simulink model "controller_simulation"  (R2024a)
settings: Solver=ode45  StartTime=0.0  StopTime=35  FixedStep=0.01  MaxStep=0.01  RelTol=1e-3
values from neighbouring files (symbols this model uses):
  Kd = diag([40,  40,  40,  40])    [initialize.m]
  Kp = diag([500, 500, 500, 500])    [initialize.m]
  q_init = traj.Vitridat(2:5, 1)    [initialize.m]
settings Model: Creator=hason  LastModifiedBy=hason
settings DataIOCC: OutputOption=SpecifiedOutputTimes  OutputTimes=[0:0.01:35]

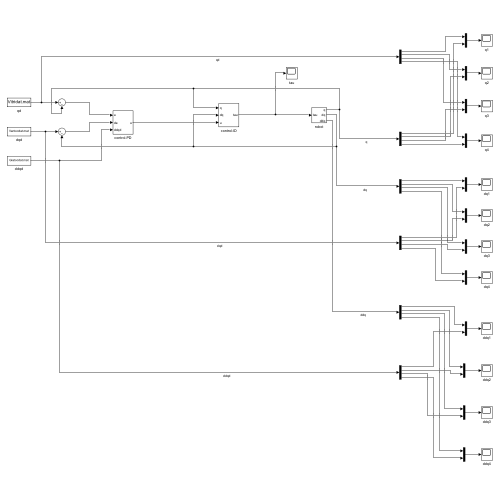
[thumbnail: Simulink's stored preview of the top-level diagram]
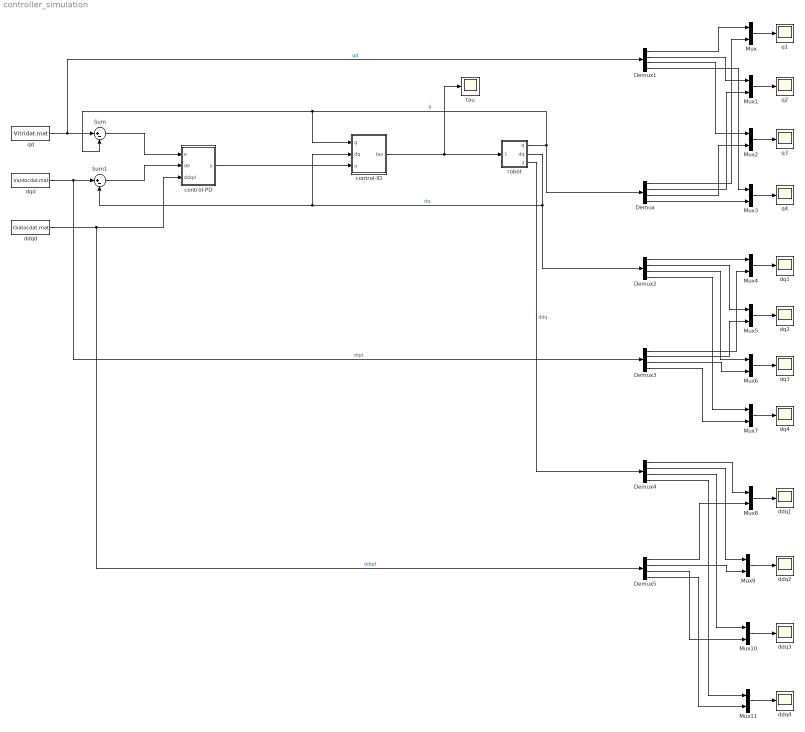
== system controller_simulation ==
  Demux{,1..5} (6 alike) : Demux
  Mux{,1..11} (12 alike) : Mux  Inputs=2
  Sum : Sum  Inputs=|+-
  Sum1 : Sum  Inputs=|+-
  control-ID : Subsystem
  control-PD : Subsystem
  ddq{1..4} (4 alike) : Scope
  ddqd : FromFile  FileName=Giatocdat.mat  SampleTime=0.01  ExtrapolationBeforeFirstDataPoint=Hold first value  InterpolationWithinTimeRange=Zero order hold  ExtrapolationAfterLastDataPoint=Ground value
  dq{1..4} (4 alike) : Scope
  dqd : FromFile  FileName=Vantocdat.mat  SampleTime=0.01  ExtrapolationBeforeFirstDataPoint=Hold first value  ExtrapolationAfterLastDataPoint=Ground value
  q{1..4} (4 alike) : Scope
  qd : FromFile  FileName=Vitridat.mat  SampleTime=0.01  ExtrapolationBeforeFirstDataPoint=Hold first value  ExtrapolationAfterLastDataPoint=Hold last value
  robot : Subsystem
  tau : Scope
  wires:
  qd/1 -> Sum/1, Demux1/1  "qd"
  dqd/1 -> Demux3/1, Sum1/1  "dqd"
  Sum/1 -> control-PD/1(e)
  Sum1/1 -> control-PD/2(de)
  ddqd/1 -> Demux5/1, control-PD/3(ddqd)  "ddqd"
  robot/1(q) -> Demux/1, control-ID/1(q), Sum/2  "q"
  control-PD/1(u) -> control-ID/3(u)
  control-ID/1(tau) -> tau/1, robot/1(tau)
  Demux1/1 -> Mux/1
  Mux/1 -> q1/1
  Mux3/1 -> q4/1
  Mux2/1 -> q3/1
  Mux1/1 -> q2/1
  Demux/1 -> Mux/2
  Demux1/2 -> Mux1/1
  Demux/2 -> Mux1/2
  Demux1/3 -> Mux2/1
  Demux/3 -> Mux2/2
  Demux1/4 -> Mux3/1
  Demux/4 -> Mux3/2
  robot/2(dq) -> Demux2/1, control-ID/2(dq), Sum1/2  "dq"
  Mux4/1 -> dq1/1
  Demux2/1 -> Mux4/1
  Demux3/1 -> Mux4/2
  Mux5/1 -> dq2/1
  Mux6/1 -> dq3/1
  Mux7/1 -> dq4/1
  Demux2/2 -> Mux5/1
  Demux3/2 -> Mux5/2
  Demux2/3 -> Mux6/1
  Demux3/3 -> Mux6/2
  Demux2/4 -> Mux7/1
  Demux3/4 -> Mux7/2
  robot/3(ddq) -> Demux4/1  "ddq"
  Mux8/1 -> ddq1/1
  Mux9/1 -> ddq2/1
  Mux10/1 -> ddq3/1
  Mux11/1 -> ddq4/1
  Demux4/1 -> Mux8/1
  Demux4/2 -> Mux9/1
  Demux4/3 -> Mux10/1
  Demux4/4 -> Mux11/1
  Demux5/1 -> Mux8/2
  Demux5/2 -> Mux9/2
  Demux5/3 -> Mux10/2
  Demux5/4 -> Mux11/2

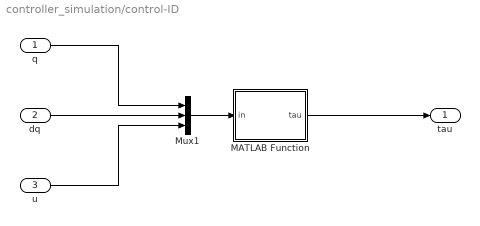
== system controller_simulation/control-ID ==
  q : Inport
  dq : Inport  Port=2
  u : Inport  Port=3
  MATLAB Function : MATLAB Function  TreatAsAtomicUnit=on
  Mux1 : Mux  Inputs=3
  tau : Outport
  wires:
  Mux1/1 -> MATLAB Function/1(in)
  q/1 -> Mux1/1
  MATLAB Function/1(tau) -> tau/1
  u/1 -> Mux1/3
  dq/1 -> Mux1/2

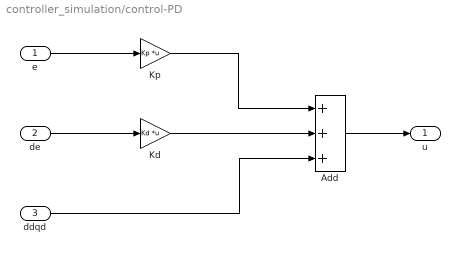
== system controller_simulation/control-PD ==
  e : Inport
  de : Inport  Port=2
  ddqd : Inport  Port=3
  Add : Sum  Inputs=+++
  Kd : Gain  Gain=Kd  Multiplication=Matrix(K*u)
  Kp : Gain  Gain=Kp  Multiplication=Matrix(K*u)
  u : Outport
  wires:
  Add/1 -> u/1
  Kp/1 -> Add/1
  ddqd/1 -> Add/3
  Kd/1 -> Add/2
  de/1 -> Kd/1
  e/1 -> Kp/1

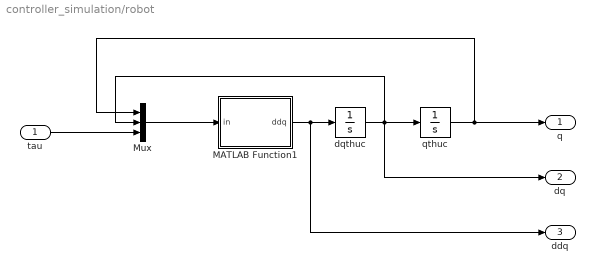
== system controller_simulation/robot ==
  tau : Inport
  MATLAB Function1 : MATLAB Function  TreatAsAtomicUnit=on
  Mux : Mux  Inputs=3
  dqthuc : Integrator  InitialCondition=[0; 0; 0; 0]
  qthuc : Integrator  InitialCondition=q_init
  q : Outport
  dq : Outport  Port=2
  ddq : Outport  Port=3
  wires:
  qthuc/1 -> q/1, Mux/1
  tau/1 -> Mux/3
  dqthuc/1 -> dq/1, qthuc/1, Mux/2
  Mux/1 -> MATLAB Function1/1(in)
  MATLAB Function1/1(ddq) -> ddq/1, dqthuc/1

== matlab function controller_simulation/control-ID/MATLAB Function ==
  data: in input; tau output; p parameter
function tau = ID_controller(in, p)
    % Input: in = [q1; q2; q3; q4; dq1; dq2; dq3; dq4; u1; u2; u3; u4]
    % Output: tau = [tau1; tau2; tau3; tau4]

    % --- 0. Khởi tạo kích thước đầu ra (Bắt buộc để cổng ra hiện số 4) ---
    tau = zeros(4,1);
    
    % --- 1. Tách biến từ input Simulink (Đổi sang dq để tránh trùng tên) ---
    q1  = in(1);  q2  = in(2);  q3  = in(3);  q4  = in(4);
    dq1 = in(5);  dq2 = in(6);  dq3 = in(7);  dq4 = in(8);
    u   = in(9:12); % u là tín hiệu gia tốc lệnh (Size 4x1)
    
    % --- 2. Khai báo biến global ---
    g = p.g; a2 = p.a2; d3 = p.d3; d4 = p.d4;
    m1 = p.m1; m2 = p.m2; m3 = p.m3; m4 = p.m4;
    xc1 = p.xc1; xc2 = p.xc2; xc3 = p.xc3; xc4 = p.xc4; % THÊM p.xc1 vào đây
    yc1 = p.yc1; yc3 = p.yc3; yc4 = p.yc4;              % Đã có p.yc1
    zc2 = p.zc2; zc3 = p.zc3; zc4 = p.zc4;
    Ixx3 = p.Ixx3; Ixx4 = p.Ixx4; Iyy2 = p.Iyy2; Iyy3 = p.Iyy3; Iyy4 = p.Iyy4; 
    Izz1 = p.Izz1; Izz3 = p.Izz3; Izz4 = p.Izz4;
    Ixy3 = p.Ixy3; Ixy4 = p.Ixy4; Ixz3 = p.Ixz3; Ixz4 = p.Ixz4; Iyz3 = p.Iyz3; Iyz4 = p.Iyz4;
    
    % --- 3. Tính toán Ma trận M, C, G (Copy từ robot_model) ---
    Cq1 = cos(q1); Sq1 = sin(q1);
    Cq3 = cos(q3); Sq3 = sin(q3);
    Cq4 = cos(q4); Sq4 = sin(q4);
    
    M = zeros(4,4);
    
    M(1,1) = (((-xc4^2+yc4^2)*m4+Ixx4)*Cq4^2+2*Sq4*(m4*xc4*yc4-Ixy4)*Cq4+Iyy4*Sq4^2+(d4+zc4)^2*m4+m3*zc3^2+Ixx3)*Cq3^2+2*(((-xc4*(d4+zc4)*m4+Ixz4)*Cq4+(yc4*(d4+zc4)*m4-Iyz4)*Sq4-m3*xc3*zc3+Ixz3)*Sq3+((d4+zc4)*m4+m3*zc3)*a2)*Cq3+(m3*xc3^2+m4*yc4^2+Izz3+Izz4)*Sq3^2-2*a2*(xc4*m4*Cq4-yc4*Sq4*m4+xc3*m3)*Sq3+2*d3*m4*yc4*Cq4+2*d3*m4*xc4*Sq4+(a2^2+d3^2+xc4^2)*m4+(m2+m3)*a2^2+2*a2*m2*xc2+(d3+yc3)^2*m3+(xc2^2+zc2^2)*m2+(xc1^2+yc1^2)*m1+Iyy2+Izz1;
    M(1,2) = 0;
    M(1,3) = (2*(-m4*xc4*yc4+Ixy4)*Cq4^2+(((-xc4^2+yc4^2)*m4+Ixx4-Iyy4)*Sq4-d3*m4*xc4)*Cq4+d3*yc4*Sq4*m4-d3*m3*xc3+m4*xc4*yc4-m3*xc3*yc3+Ixy3-Ixy4)*Cq3-((yc4*(d4+zc4)*m4-Iyz4)*Cq4+(xc4*(d4+zc4)*m4-Ixz4)*Sq4+d3*(d4+zc4)*m4+d3*m3*zc3+m3*yc3*zc3-Iyz3)*Sq3;
    M(1,4) = ((-xc4*(d4+zc4)*m4+Ixz4)*Cq4-(-yc4*(d4+zc4)*m4+Iyz4)*Sq4)*Cq3-m4*(-d3*yc4*Sq3+a2*xc4)*Cq4+(d3*m4*xc4*Sq4+(xc4^2+yc4^2)*m4+Izz4)*Sq3+a2*m4*yc4*Sq4;
    M(2,1) = 0; M(2,2) = m2+m3+m4;
    M(2,3) = ((d4+zc4)*m4+m3*zc3)*Cq3-Sq3*(xc4*m4*Cq4-yc4*Sq4*m4+xc3*m3);
    M(2,4) = -(Sq4*xc4+Cq4*yc4)*Cq3*m4;
    M(3,1) = M(1,3); M(3,2) = M(2,3);
    M(3,3) = (m4*xc4^2+Iyy4)*Cq4^2+2*Sq4*(-m4*xc4*yc4+Ixy4)*Cq4+(m4*yc4^2+Ixx4)*Sq4^2+(d4+zc4)^2*m4+m3*xc3^2+m3*zc3^2+Iyy3;
    M(3,4) = (-yc4*(d4+zc4)*m4+Iyz4)*Cq4-(xc4*(d4+zc4)*m4-Ixz4)*Sq4;
    M(4,1) = M(1,4); M(4,2) = M(2,4); M(4,3) = M(3,4);
    M(4,4) = Izz4+(xc4^2+yc4^2)*m4;
    
    C = zeros(4,4);
    
    C(1,1) = (dq4*(m4*xc4*yc4-Ixy4)*Cq4^2+(((xc4^2-yc4^2)*m4-Ixx4+Iyy4)*dq4*Sq4-dq3*(xc4*(d4+zc4)*m4-Ixz4))*Cq4-dq4*(m4*xc4*yc4-Ixy4)*Sq4^2+dq3*(yc4*(d4+zc4)*m4-Iyz4)*Sq4-dq3*(m3*xc3*zc3-Ixz3))*Cq3^2+((dq3*((xc4^2-yc4^2)*m4-Ixx4)*Cq4^2+(-2*dq3*(m4*xc4*yc4-Ixy4)*Sq4+(yc4*(d4+zc4)*m4-Iyz4)*dq4)*Cq4-Iyy4*Sq4^2*dq3+(xc4*(d4+zc4)*m4-Ixz4)*dq4*Sq4+((yc4+zc4+d4)*(yc4-zc4-d4)*m4+(xc3^2-zc3^2)*m3-Ixx3+Izz3+Izz4)*dq3)*Sq3-a2*dq3*(xc4*m4*Cq4-yc4*Sq4*m4+xc3*m3))*Cq3+((xc4*(d4+zc4)*m4-Ixz4)*Cq4+(-yc4*(d4+zc4)*m4+Iyz4)*Sq4+m3*xc3*zc3-Ixz3)*dq3*Sq3^2+a2*(yc4*m4*dq4*Cq4+xc4*Sq4*m4*dq4-dq3*((d4+zc4)*m4+m3*zc3))*Sq3+d3*m4*dq4*(Cq4*xc4-Sq4*yc4);
    C(1,3) = -((xc4*(d4+zc4)*m4-Ixz4)*Cq4+(-yc4*(d4+zc4)*m4+Iyz4)*Sq4+m3*xc3*zc3-Ixz3)*dq1*Cq3^2+1/2*(2*(((xc4^2-yc4^2)*m4-Ixx4)*Cq4^2-2*Sq4*(m4*xc4*yc4-Ixy4)*Cq4-Iyy4*Sq4^2+(yc4+zc4+d4)*(yc4-zc4-d4)*m4+(xc3^2-zc3^2)*m3-Ixx3+Izz3+Izz4)*dq1*Sq3-((xc4^2-yc4^2)*m4-Ixx4+Iyy4)*dq4*Cq4^2+2*(2*dq4*(m4*xc4*yc4-Ixy4)*Sq4+(-a2*xc4*dq1+(-(d4+zc4)*dq3+dq4*d3)*yc4)*m4+Iyz4*dq3)*Cq4+((xc4^2-yc4^2)*m4-Ixx4+Iyy4)*dq4*Sq4^2+2*((a2*yc4*dq1+(-(d4+zc4)*dq3+dq4*d3)*xc4)*m4+Ixz4*dq3)*Sq4+(-2*d3*(d4+zc4)*dq3+dq4*(xc4^2+yc4^2))*m4-2*a2*m3*dq1*xc3+2*(-zc3*(d3+yc3)*m3+Iyz3)*dq3+Izz4*dq4)*Cq3-Sq3*(-((xc4*(d4+zc4)*m4-Ixz4)*Cq4+(-yc4*(d4+zc4)*m4+Iyz4)*Sq4+m3*xc3*zc3-Ixz3)*dq1*Sq3-2*dq3*(m4*xc4*yc4-Ixy4)*Cq4^2-dq3*(((xc4^2-yc4^2)*m4-Ixx4+Iyy4)*Sq4+d3*m4*xc4)*Cq4+Sq4*d3*m4*dq3*yc4+(a2*(d4+zc4)*dq1+xc4*yc4*dq3)*m4+a2*m3*dq1*zc3-(xc3*(d3+yc3)*m3-Ixy3+Ixy4)*dq3);
    C(1,4) = (Cq4^2*(m4*xc4*yc4-Ixy4)+((xc4^2-yc4^2)*m4-Ixx4+Iyy4)*Sq4*Cq4-Sq4^2*(m4*xc4*yc4-Ixy4))*dq1*Cq3^2+1/2*(-((xc4^2-yc4^2)*m4-Ixx4+Iyy4)*dq3*Cq4^2+2*(2*dq3*(m4*xc4*yc4-Ixy4)*Sq4+(yc4*(d4+zc4)*m4-Iyz4)*dq1*Sq3+yc4*(d3*dq3+dq4*(d4+zc4))*m4-Iyz4*dq4)*Cq4+((xc4^2-yc4^2)*m4-Ixx4+Iyy4)*dq3*Sq4^2+2*((xc4*(d4+zc4)*m4-Ixz4)*dq1*Sq3+xc4*(d3*dq3+dq4*(d4+zc4))*m4-Ixz4*dq4)*Sq4+dq3*(Izz4+(xc4^2+yc4^2)*m4))*Cq3+m4*(((a2*dq1*yc4+d3*dq4*xc4)*Sq3+a2*yc4*dq4+xc4*d3*dq1)*Cq4+((a2*dq1*xc4-d3*dq4*yc4)*Sq3+a2*xc4*dq4-yc4*d3*dq1)*Sq4);
    C(2,3) = (yc4*m4*dq4*Cq4+xc4*Sq4*m4*dq4-dq3*((d4+zc4)*m4+m3*zc3))*Sq3+Cq3*dq3*(-xc4*m4*Cq4+yc4*Sq4*m4-xc3*m3);
    C(2,4) = m4*(dq4*(-Cq4*xc4+Sq4*yc4)*Cq3+dq3*(Sq4*xc4+Cq4*yc4)*Sq3);
    C(3,1) = ((xc4*(d4+zc4)*m4-Ixz4)*Cq4+(-yc4*(d4+zc4)*m4+Iyz4)*Sq4+m3*xc3*zc3-Ixz3)*dq1*Cq3^2+1/2*(-2*(((xc4^2-yc4^2)*m4-Ixx4)*Cq4^2-2*Sq4*(m4*xc4*yc4-Ixy4)*Cq4-Iyy4*Sq4^2+(yc4+zc4+d4)*(yc4-zc4-d4)*m4+(xc3^2-zc3^2)*m3-Ixx3+Izz3+Izz4)*dq1*Sq3-((xc4^2-yc4^2)*m4-Ixx4+Iyy4)*dq4*Cq4^2+2*(2*dq4*(m4*xc4*yc4-Ixy4)*Sq4+a2*m4*dq1*xc4)*Cq4+((xc4^2-yc4^2)*m4-Ixx4+Iyy4)*dq4*Sq4^2-2*Sq4*a2*m4*dq1*yc4+2*a2*m3*dq1*xc3-(Izz4+(xc4^2+yc4^2)*m4)*dq4)*Cq3+(-((xc4*(d4+zc4)*m4-Ixz4)*Cq4+(-yc4*(d4+zc4)*m4+Iyz4)*Sq4+m3*xc3*zc3-Ixz3)*dq1*Sq3-(xc4*(d4+zc4)*m4-Ixz4)*dq4*Cq4+(yc4*(d4+zc4)*m4-Iyz4)*dq4*Sq4+dq1*a2*((d4+zc4)*m4+m3*zc3))*Sq3;
    C(3,3) = -1/2*(((xc4^2-yc4^2)*m4-Ixx4+Iyy4)*sin(2*q4)+2*cos(2*q4)*(m4*xc4*yc4-Ixy4))*dq4;
    C(3,4) = (dq1*(-m4*xc4^2+Ixx4-Iyy4)*Cq3+2*dq3*(-m4*xc4*yc4+Ixy4))*Cq4^2+((-2*dq1*(-m4*xc4*yc4+Ixy4)*Cq3+dq3*((-xc4^2+yc4^2)*m4+Ixx4-Iyy4))*Sq4-(dq4+Sq3*dq1)*(xc4*(d4+zc4)*m4-Ixz4))*Cq4-Cq3*Sq4^2*m4*dq1*yc4^2+(yc4*(d4+zc4)*m4-Iyz4)*(dq4+Sq3*dq1)*Sq4-1/2*dq1*(Ixx4-Iyy4+Izz4)*Cq3-dq3*(-m4*xc4*yc4+Ixy4);
    C(4,1) = ((-m4*xc4*yc4+Ixy4)*Cq4^2+((-xc4^2+yc4^2)*m4+Ixx4-Iyy4)*Sq4*Cq4+Sq4^2*(m4*xc4*yc4-Ixy4))*dq1*Cq3^2+1/2*(-((-xc4^2+yc4^2)*m4+Ixx4-Iyy4)*dq3*Cq4^2+2*(-2*dq3*(m4*xc4*yc4-Ixy4)*Sq4-(yc4*(d4+zc4)*m4-Iyz4)*dq1*Sq3)*Cq4+((-xc4^2+yc4^2)*m4+Ixx4-Iyy4)*dq3*Sq4^2-2*(xc4*(d4+zc4)*m4-Ixz4)*Sq3*dq1*Sq4+dq3*(Izz4+(xc4^2+yc4^2)*m4))*Cq3+(((xc4*(d4+zc4)*dq3-a2*yc4*dq1)*m4-Ixz4*dq3)*Sq3-d3*m4*dq1*xc4)*Cq4-Sq4*(((yc4*(d4+zc4)*dq3+a2*xc4*dq1)*m4-Iyz4*dq3)*Sq3-d3*m4*dq1*yc4);
    C(4,3) = (-dq1*(-m4*xc4^2+Ixx4-Iyy4)*Cq3-2*dq3*(-m4*xc4*yc4+Ixy4))*Cq4^2+((2*dq1*(-m4*xc4*yc4+Ixy4)*Cq3-dq3*((-xc4^2+yc4^2)*m4+Ixx4-Iyy4))*Sq4+(xc4*(d4+zc4)*m4-Ixz4)*dq1*Sq3)*Cq4+Cq3*Sq4^2*m4*dq1*yc4^2-dq1*(yc4*(d4+zc4)*m4-Iyz4)*Sq3*Sq4+1/2*dq1*(Ixx4-Iyy4+Izz4)*Cq3+dq3*(-m4*xc4*yc4+Ixy4);
    
    G = zeros(4,1);
    G(2,1) = g*(m2+m3+m4);
    G(3,1) = g*(((d4+zc4)*m4+m3*zc3)*Cq3-Sq3*(xc4*m4*Cq4-yc4*Sq4*m4+xc3*m3));
    G(4,1) = -m4*(Sq4*xc4+Cq4*yc4)*Cq3*g;
    
    % --- 4. Luật điều khiển IDPD (Computed Torque) ---
    dq_vector = [dq1; dq2; dq3; dq4]; % Vector cột 4x1
    
    % Phép toán: (4x4)*(4x1) + (4x4)*(4x1) + (4x1) = (4x1)
    tau = M * u + C * dq_vector + G;
end

== matlab function controller_simulation/robot/MATLAB Function1 ==
  data: in input; ddq output; p parameter
function ddq = fcn(in, p)
    % Input: in = [q1, q2, q3, q4, dq1, dq2, dq3, dq4, tau1, tau2, tau3, tau4]
    
    % --- 0. Khởi tạo kích thước đầu ra (Bắt buộc để cổng ra hiện số 4) ---
    ddq = zeros(4,1);
    
    % --- 1. Tách tín hiệu (Đổi sang dq để tránh trùng tên biến) ---
    q = in(1:4); 
    dq_vec = in(5:8); % Vector vận tốc khớp thực tế (4x1)
    tau = in(9:12);   % Vector mô-men xoắn từ bộ điều khiển đưa vào (4x1)
    
    q1=q(1);   q2=q(2);   q3=q(3);   q4=q(4);
    dq1=dq_vec(1); dq2=dq_vec(2); dq3=dq_vec(3); dq4=dq_vec(4);
    
    % --- 2. Khai báo biến toàn cục ---
    g = p.g; a2 = p.a2; d3 = p.d3; d4 = p.d4;
    m1 = p.m1; m2 = p.m2; m3 = p.m3; m4 = p.m4;
    xc1 = p.xc1; xc2 = p.xc2; xc3 = p.xc3; xc4 = p.xc4; % THÊM p.xc1 vào đây
    yc1 = p.yc1; yc3 = p.yc3; yc4 = p.yc4;              % Đã có p.yc1
    zc2 = p.zc2; zc3 = p.zc3; zc4 = p.zc4;
    Ixx3 = p.Ixx3; Ixx4 = p.Ixx4; Iyy2 = p.Iyy2; Iyy3 = p.Iyy3; Iyy4 = p.Iyy4; 
    Izz1 = p.Izz1; Izz3 = p.Izz3; Izz4 = p.Izz4;
    Ixy3 = p.Ixy3; Ixy4 = p.Ixy4; Ixz3 = p.Ixz3; Ixz4 = p.Ixz4; Iyz3 = p.Iyz3; Iyz4 = p.Iyz4;
    
    % --- 3. Tính toán Ma trận M, C, G ---
    Cq1 = cos(q1); Sq1 = sin(q1); Cq3 = cos(q3); Sq3 = sin(q3); Cq4 = cos(q4); Sq4 = sin(q4);
    
    % ---- Ma tran khoi luong M(q) ----
    M = zeros(4,4);
    M(1,1) = (((-xc4^2+yc4^2)*m4+Ixx4)*Cq4^2+2*Sq4*(m4*xc4*yc4-Ixy4)*Cq4+Iyy4*Sq4^2+(d4+zc4)^2*m4+m3*zc3^2+Ixx3)*Cq3^2+2*(((-xc4*(d4+zc4)*m4+Ixz4)*Cq4+(yc4*(d4+zc4)*m4-Iyz4)*Sq4-m3*xc3*zc3+Ixz3)*Sq3+((d4+zc4)*m4+m3*zc3)*a2)*Cq3+(m3*xc3^2+m4*yc4^2+Izz3+Izz4)*Sq3^2-2*a2*(xc4*m4*Cq4-yc4*Sq4*m4+xc3*m3)*Sq3+2*d3*m4*yc4*Cq4+2*d3*m4*xc4*Sq4+(a2^2+d3^2+xc4^2)*m4+(m2+m3)*a2^2+2*a2*m2*xc2+(d3+yc3)^2*m3+(xc2^2+zc2^2)*m2+(xc1^2+yc1^2)*m1+Iyy2+Izz1;
    M(1,2) = 0;
    M(1,3) = (2*(-m4*xc4*yc4+Ixy4)*Cq4^2+(((-xc4^2+yc4^2)*m4+Ixx4-Iyy4)*Sq4-d3*m4*xc4)*Cq4+d3*yc4*Sq4*m4-d3*m3*xc3+m4*xc4*yc4-m3*xc3*yc3+Ixy3-Ixy4)*Cq3-((yc4*(d4+zc4)*m4-Iyz4)*Cq4+(xc4*(d4+zc4)*m4-Ixz4)*Sq4+d3*(d4+zc4)*m4+d3*m3*zc3+m3*yc3*zc3-Iyz3)*Sq3;
    M(1,4) = ((-xc4*(d4+zc4)*m4+Ixz4)*Cq4-(-yc4*(d4+zc4)*m4+Iyz4)*Sq4)*Cq3-m4*(-d3*yc4*Sq3+a2*xc4)*Cq4+(d3*m4*xc4*Sq4+(xc4^2+yc4^2)*m4+Izz4)*Sq3+a2*m4*yc4*Sq4;
    M(2,1) = 0;
    M(2,2) = m2+m3+m4;
    M(2,3) = ((d4+zc4)*m4+m3*zc3)*Cq3-Sq3*(xc4*m4*Cq4-yc4*Sq4*m4+xc3*m3);
    M(2,4) = -(Sq4*xc4+Cq4*yc4)*Cq3*m4;
    M(3,1) = M(1,3);
    M(3,2) = M(2,3);
    M(3,3) = (m4*xc4^2+Iyy4)*Cq4^2+2*Sq4*(-m4*xc4*yc4+Ixy4)*Cq4+(m4*yc4^2+Ixx4)*Sq4^2+(d4+zc4)^2*m4+m3*xc3^2+m3*zc3^2+Iyy3;
    M(3,4) = (-yc4*(d4+zc4)*m4+Iyz4)*Cq4-(xc4*(d4+zc4)*m4-Ixz4)*Sq4;
    M(4,1) = M(1,4);
    M(4,2) = M(2,4);
    M(4,3) = M(3,4);
    M(4,4) = Izz4+(xc4^2+yc4^2)*m4;
    
    % ---- Ma tran Coriolis C(q,dq) ----
    C = zeros(4,4);
    C(1,1) = (dq4*(m4*xc4*yc4-Ixy4)*Cq4^2+(((xc4^2-yc4^2)*m4-Ixx4+Iyy4)*dq4*Sq4-dq3*(xc4*(d4+zc4)*m4-Ixz4))*Cq4-dq4*(m4*xc4*yc4-Ixy4)*Sq4^2+dq3*(yc4*(d4+zc4)*m4-Iyz4)*Sq4-dq3*(m3*xc3*zc3-Ixz3))*Cq3^2+((dq3*((xc4^2-yc4^2)*m4-Ixx4)*Cq4^2+(-2*dq3*(m4*xc4*yc4-Ixy4)*Sq4+(yc4*(d4+zc4)*m4-Iyz4)*dq4)*Cq4-Iyy4*Sq4^2*dq3+(xc4*(d4+zc4)*m4-Ixz4)*dq4*Sq4+((yc4+zc4+d4)*(yc4-zc4-d4)*m4+(xc3^2-zc3^2)*m3-Ixx3+Izz3+Izz4)*dq3)*Sq3-a2*dq3*(xc4*m4*Cq4-yc4*Sq4*m4+xc3*m3))*Cq3+((xc4*(d4+zc4)*m4-Ixz4)*Cq4+(-yc4*(d4+zc4)*m4+Iyz4)*Sq4+m3*xc3*zc3-Ixz3)*dq3*Sq3^2+a2*(yc4*m4*dq4*Cq4+xc4*Sq4*m4*dq4-dq3*((d4+zc4)*m4+m3*zc3))*Sq3+d3*m4*dq4*(Cq4*xc4-Sq4*yc4);
    C(1,2) = 0;
    C(1,3) = -((xc4*(d4+zc4)*m4-Ixz4)*Cq4+(-yc4*(d4+zc4)*m4+Iyz4)*Sq4+m3*xc3*zc3-Ixz3)*dq1*Cq3^2+1/2*(2*(((xc4^2-yc4^2)*m4-Ixx4)*Cq4^2-2*Sq4*(m4*xc4*yc4-Ixy4)*Cq4-Iyy4*Sq4^2+(yc4+zc4+d4)*(yc4-zc4-d4)*m4+(xc3^2-zc3^2)*m3-Ixx3+Izz3+Izz4)*dq1*Sq3-((xc4^2-yc4^2)*m4-Ixx4+Iyy4)*dq4*Cq4^2+2*(2*dq4*(m4*xc4*yc4-Ixy4)*Sq4+(-a2*xc4*dq1+(-(d4+zc4)*dq3+dq4*d3)*yc4)*m4+Iyz4*dq3)*Cq4+((xc4^2-yc4^2)*m4-Ixx4+Iyy4)*dq4*Sq4^2+2*((a2*yc4*dq1+(-(d4+zc4)*dq3+dq4*d3)*xc4)*m4+Ixz4*dq3)*Sq4+(-2*d3*(d4+zc4)*dq3+dq4*(xc4^2+yc4^2))*m4-2*a2*m3*dq1*xc3+2*(-zc3*(d3+yc3)*m3+Iyz3)*dq3+Izz4*dq4)*Cq3-Sq3*(-((xc4*(d4+zc4)*m4-Ixz4)*Cq4+(-yc4*(d4+zc4)*m4+Iyz4)*Sq4+m3*xc3*zc3-Ixz3)*dq1*Sq3-2*dq3*(m4*xc4*yc4-Ixy4)*Cq4^2-dq3*(((xc4^2-yc4^2)*m4-Ixx4+Iyy4)*Sq4+d3*m4*xc4)*Cq4+Sq4*d3*m4*dq3*yc4+(a2*(d4+zc4)*dq1+xc4*yc4*dq3)*m4+a2*m3*dq1*zc3-(xc3*(d3+yc3)*m3-Ixy3+Ixy4)*dq3);
    C(1,4) = (Cq4^2*(m4*xc4*yc4-Ixy4)+((xc4^2-yc4^2)*m4-Ixx4+Iyy4)*Sq4*Cq4-Sq4^2*(m4*xc4*yc4-Ixy4))*dq1*Cq3^2+1/2*(-((xc4^2-yc4^2)*m4-Ixx4+Iyy4)*dq3*Cq4^2+2*(2*dq3*(m4*xc4*yc4-Ixy4)*Sq4+(yc4*(d4+zc4)*m4-Iyz4)*dq1*Sq3+yc4*(d3*dq3+dq4*(d4+zc4))*m4-Iyz4*dq4)*Cq4+((xc4^2-yc4^2)*m4-Ixx4+Iyy4)*dq3*Sq4^2+2*((xc4*(d4+zc4)*m4-Ixz4)*dq1*Sq3+xc4*(d3*dq3+dq4*(d4+zc4))*m4-Ixz4*dq4)*Sq4+dq3*(Izz4+(xc4^2+yc4^2)*m4))*Cq3+m4*(((a2*dq1*yc4+d3*dq4*xc4)*Sq3+a2*yc4*dq4+xc4*d3*dq1)*Cq4+((a2*dq1*xc4-d3*dq4*yc4)*Sq3+a2*xc4*dq4-yc4*d3*dq1)*Sq4);
    C(2,1) = 0;
    C(2,2) = 0;
    C(2,3) = (yc4*m4*dq4*Cq4+xc4*Sq4*m4*dq4-dq3*((d4+zc4)*m4+m3*zc3))*Sq3+Cq3*dq3*(-xc4*m4*Cq4+yc4*Sq4*m4-xc3*m3);
    C(2,4) = m4*(dq4*(-Cq4*xc4+Sq4*yc4)*Cq3+dq3*(Sq4*xc4+Cq4*yc4)*Sq3);
    C(3,1) = ((xc4*(d4+zc4)*m4-Ixz4)*Cq4+(-yc4*(d4+zc4)*m4+Iyz4)*Sq4+m3*xc3*zc3-Ixz3)*dq1*Cq3^2+1/2*(-2*(((xc4^2-yc4^2)*m4-Ixx4)*Cq4^2-2*Sq4*(m4*xc4*yc4-Ixy4)*Cq4-Iyy4*Sq4^2+(yc4+zc4+d4)*(yc4-zc4-d4)*m4+(xc3^2-zc3^2)*m3-Ixx3+Izz3+Izz4)*dq1*Sq3-((xc4^2-yc4^2)*m4-Ixx4+Iyy4)*dq4*Cq4^2+2*(2*dq4*(m4*xc4*yc4-Ixy4)*Sq4+a2*m4*dq1*xc4)*Cq4+((xc4^2-yc4^2)*m4-Ixx4+Iyy4)*dq4*Sq4^2-2*Sq4*a2*m4*dq1*yc4+2*a2*m3*dq1*xc3-(Izz4+(xc4^2+yc4^2)*m4)*dq4)*Cq3+(-((xc4*(d4+zc4)*m4-Ixz4)*Cq4+(-yc4*(d4+zc4)*m4+Iyz4)*Sq4+m3*xc3*zc3-Ixz3)*dq1*Sq3-(xc4*(d4+zc4)*m4-Ixz4)*dq4*Cq4+(yc4*(d4+zc4)*m4-Iyz4)*dq4*Sq4+dq1*a2*((d4+zc4)*m4+m3*zc3))*Sq3;
    C(3,2) = 0;
    C(3,3) = -1/2*(((xc4^2-yc4^2)*m4-Ixx4+Iyy4)*sin(2*q4)+2*cos(2*q4)*(m4*xc4*yc4-Ixy4))*dq4;
    C(3,4) = (dq1*(-m4*xc4^2+Ixx4-Iyy4)*Cq3+2*dq3*(-m4*xc4*yc4+Ixy4))*Cq4^2+((-2*dq1*(-m4*xc4*yc4+Ixy4)*Cq3+dq3*((-xc4^2+yc4^2)*m4+Ixx4-Iyy4))*Sq4-(dq4+Sq3*dq1)*(xc4*(d4+zc4)*m4-Ixz4))*Cq4-Cq3*Sq4^2*m4*dq1*yc4^2+(yc4*(d4+zc4)*m4-Iyz4)*(dq4+Sq3*dq1)*Sq4-1/2*dq1*(Ixx4-Iyy4+Izz4)*Cq3-dq3*(-m4*xc4*yc4+Ixy4);
    C(4,1) = ((-m4*xc4*yc4+Ixy4)*Cq4^2+((-xc4^2+yc4^2)*m4+Ixx4-Iyy4)*Sq4*Cq4+Sq4^2*(m4*xc4*yc4-Ixy4))*dq1*Cq3^2+1/2*(-((-xc4^2+yc4^2)*m4+Ixx4-Iyy4)*dq3*Cq4^2+2*(-2*dq3*(m4*xc4*yc4-Ixy4)*Sq4-(yc4*(d4+zc4)*m4-Iyz4)*dq1*Sq3)*Cq4+((-xc4^2+yc4^2)*m4+Ixx4-Iyy4)*dq3*Sq4^2-2*(xc4*(d4+zc4)*m4-Ixz4)*Sq3*dq1*Sq4+dq3*(Izz4+(xc4^2+yc4^2)*m4))*Cq3+(((xc4*(d4+zc4)*dq3-a2*yc4*dq1)*m4-Ixz4*dq3)*Sq3-d3*m4*dq1*xc4)*Cq4-Sq4*(((yc4*(d4+zc4)*dq3+a2*xc4*dq1)*m4-Iyz4*dq3)*Sq3-d3*m4*dq1*yc4);
    C(4,2) = 0;
    C(4,3) = (-dq1*(-m4*xc4^2+Ixx4-Iyy4)*Cq3-2*dq3*(-m4*xc4*yc4+Ixy4))*Cq4^2+((2*dq1*(-m4*xc4*yc4+Ixy4)*Cq3-dq3*((-xc4^2+yc4^2)*m4+Ixx4-Iyy4))*Sq4+(xc4*(d4+zc4)*m4-Ixz4)*dq1*Sq3)*Cq4+Cq3*Sq4^2*m4*dq1*yc4^2-dq1*(yc4*(d4+zc4)*m4-Iyz4)*Sq3*Sq4+1/2*dq1*(Ixx4-Iyy4+Izz4)*Cq3+dq3*(-m4*xc4*yc4+Ixy4);
    C(4,4) = 0;
    
    % ---- Vecto trong luc G(q) ----
    G = zeros(4,1);
    G(1,1) = 0;
    G(2,1) = g*(m2+m3+m4);
    G(3,1) = g*(((d4+zc4)*m4+m3*zc3)*Cq3-Sq3*(xc4*m4*Cq4-yc4*Sq4*m4+xc3*m3));
    G(4,1) = -m4*(Sq4*xc4+Cq4*yc4)*Cq3*g;
    
    % --- 4. Giải phương trình vi phân (Tính gia tốc khớp thực tế) ---
    % Phép toán: (4x4) \ ( (4x1) - (4x4)*(4x1) - (4x1) ) = (4x1)
    ddq = M \ (tau - C * dq_vec - G);
end
